simulink model "Appl_HeatFault_CtrlModel"  (R2018b)
settings: configuration reference "CodeConfig_10_ms" (kept outside this file)
undefined symbols (not defined in the file): CAL_CmdOpenTime, CAL_CmdShortTime, CAL_NTCOpenTime, CAL_NTCOverTime, CAL_NTCShortTime, CAL_NTCWaitTime, D_HEATFALUT_CmdOpenLoad, D_HEATFALUT_CmdOpenLoad_W, D_HEATFALUT_CmdShortToGnd, D_HEATFALUT_NtcMax, D_HEATFALUT_NtcMin, D_HEATFALUT_NtcOpenLoad, D_HEATFALUT_NtcShortToGnd, FALSE, TRUE
libraries: DareLib x32, simulink x1
(part 1 of 2)
settings Model: Creator=Administrator  LastModifiedBy=Administrator
settings ConfigSetRef: SourceLocation=Base Workspace

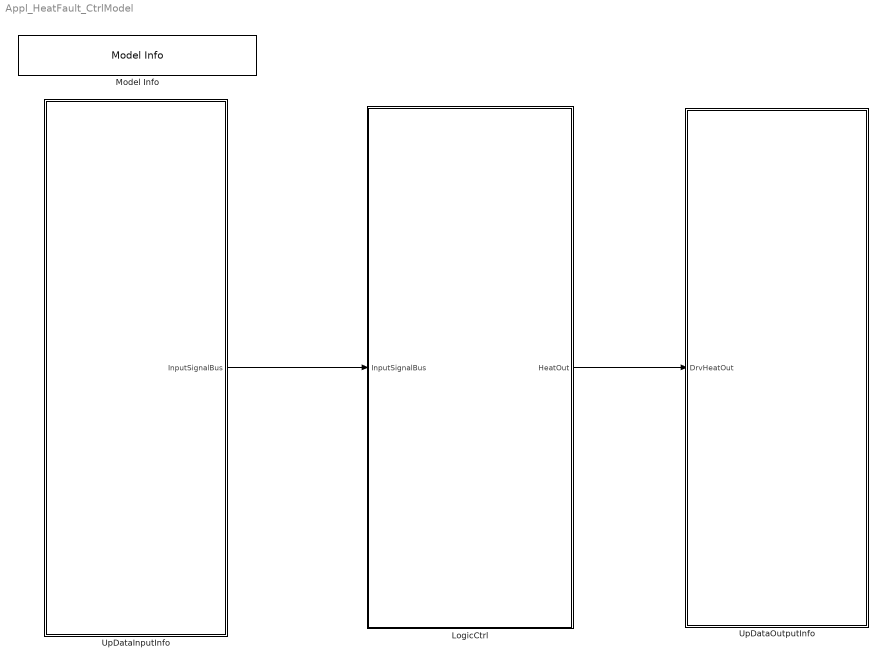
== system Appl_HeatFault_CtrlModel ==
  LogicCtrl : Subsystem  Priority=2  TreatAsAtomicUnit=on
      settings: RTWSystemCode=Nonreusable function  RTWFcnNameOpts=Use subsystem name
  Model Info : simulink/Model-Wide Utilities/Model Info  Frame=on  DisplayStringWithTags=Version：%<ModelVersion>  HorizontalTextAlignment=Center  LeftAlignmentValue=0.5
  UpDataInputInfo : Subsystem  Priority=1  TreatAsAtomicUnit=on
      settings: RTWSystemCode=Nonreusable function  RTWFcnNameOpts=Use subsystem name
  UpDataOutputInfo : Subsystem  Priority=3  TreatAsAtomicUnit=on
      settings: RTWSystemCode=Nonreusable function  RTWFcnNameOpts=Use subsystem name
  wires:
  LogicCtrl/1(HeatOut) -> UpDataOutputInfo/1(DrvHeatOut)
  UpDataInputInfo/1(InputSignalBus) -> LogicCtrl/1(InputSignalBus)

== system Appl_HeatFault_CtrlModel/LogicCtrl ==
  InputSignalBus : Inport
  Bus Selector : BusSelector  OutputSignals=Rte_SignalBus.HeatFalut_D_SimuIndex_DRHeat,Rte_SignalBus.HeatFalut_D_SimuIndex_PAHeat,Rte_SignalBus.HeatFalut_D_SimuIndex_ThirdHeat,Rte_SignalBus.HeatFalut_D_SimuIndex_DRHeatIo,Rte_SignalBus.HeatFalut_D_SimuIndex_PAHeatIo,Rte_SignalBus.HeatFalut_D_SimuIndex_ThirdHeatIo,Rte_SignalBus.HeatFalut_MemIndexDrHeatConfig,Rte_SignalBus.HeatFalut_MemIndexPaHeatConfig,Rte_SignalBus.HeatFalut_MemIndexThirdHeatConfig,Rte_SignalBus.HeatFalut_DrHeatNtcAdc,Rte_SignalBus.HeatFalut_PaHeatNtcAdc,Rte_SignalBus.HeatFalut_ThirdHeatNtcAdc,Rte_SignalBus.HeatFalut_DrHeatIsAdc,Rte_SignalBus.HeatFalut_PaHeatIsAdc,Rte_SignalBus.HeatFalut_ThirdHeatIsAdc,DrFaultType,PaFaultType,ThirdFaultType,Rte_SignalBus.HeatFalut_MemDiagDrHeatFlg,Rte_SignalBus.HeatFalut_MemDiagPaHeatFlg
  HeatDiagnoseCtrl : Subsystem  Description=加热诊断处理
      settings: AttributesFormatString=%<Description>
  MainVent_OutputLvlSts : BusCreator  Inputs=9
  HeatOut : Outport
  wires:
  InputSignalBus/1 -> Bus Selector/1  "InputSignalBus"
  MainVent_OutputLvlSts/1 -> HeatOut/1
  Bus Selector/15 -> HeatDiagnoseCtrl/15(HeatFalut_ThirdHeatIsAdc)  "<HeatFalut_ThirdHeatIsAdc>"
  Bus Selector/14 -> HeatDiagnoseCtrl/14(HeatFalut_PaHeatIsAdc)  "<HeatFalut_PaHeatIsAdc>"
  Bus Selector/13 -> HeatDiagnoseCtrl/13(HeatFalut_DrHeatIsAdc)  "<HeatFalut_DrHeatIsAdc>"
  Bus Selector/12 -> HeatDiagnoseCtrl/12(HeatFalut_ThirdHeatNtcAdc)  "<HeatFalut_ThirdHeatNtcAdc>"
  Bus Selector/11 -> HeatDiagnoseCtrl/11(HeatFalut_PaHeatNtcAdc)  "<HeatFalut_PaHeatNtcAdc>"
  Bus Selector/10 -> HeatDiagnoseCtrl/10(HeatFalut_DrHeatNtcAdc)  "<HeatFalut_DrHeatNtcAdc>"
  Bus Selector/9 -> HeatDiagnoseCtrl/9(HeatFalut_MemIndexThirdHeatConfig)  "<HeatFalut_MemIndexThirdHeatConfig>"
  Bus Selector/8 -> HeatDiagnoseCtrl/8(HeatFalut_MemIndexPaHeatConfig)  "<HeatFalut_MemIndexPaHeatConfig>"
  Bus Selector/7 -> HeatDiagnoseCtrl/7(HeatFalut_MemIndexDrHeatConfig)  "<HeatFalut_MemIndexDrHeatConfig>"
  Bus Selector/6 -> HeatDiagnoseCtrl/6(HeatFalut_D_SimuIndex_ThirdHeatIo)  "<HeatFalut_D_SimuIndex_ThirdHeatIo>"
  Bus Selector/5 -> HeatDiagnoseCtrl/5(HeatFalut_D_SimuIndex_PAHeatIo)  "<HeatFalut_D_SimuIndex_PAHeatIo>"
  Bus Selector/4 -> HeatDiagnoseCtrl/4(HeatFalut_D_SimuIndex_DRHeatIo)  "<HeatFalut_D_SimuIndex_DRHeatIo>"
  Bus Selector/3 -> HeatDiagnoseCtrl/3(HeatFalut_D_SimuIndex_ThirdHeat)  "<HeatFalut_D_SimuIndex_ThirdHeat>"
  Bus Selector/2 -> HeatDiagnoseCtrl/2(HeatFalut_D_SimuIndex_PAHeat)  "<HeatFalut_D_SimuIndex_PAHeat>"
  Bus Selector/1 -> HeatDiagnoseCtrl/1(HeatFalut_D_SimuIndex_DRHeat)  "<HeatFalut_D_SimuIndex_DRHeat>"
  HeatDiagnoseCtrl/1(HeatFault_DRHeatCmdFaultSts) -> MainVent_OutputLvlSts/1
  HeatDiagnoseCtrl/2(HeatFault_PAHeatCmdFaultSts) -> MainVent_OutputLvlSts/2
  HeatDiagnoseCtrl/3(HeatFault_ThirdHeatCmdFaultSts) -> MainVent_OutputLvlSts/3
  HeatDiagnoseCtrl/4(HeatFault_DRHeatNTCFaultSts) -> MainVent_OutputLvlSts/4
  HeatDiagnoseCtrl/5(HeatFault_PAHeatNTCFaultSts) -> MainVent_OutputLvlSts/5
  HeatDiagnoseCtrl/6(HeatFault_ThirdHeatNTCFaultSts) -> MainVent_OutputLvlSts/6
  HeatDiagnoseCtrl/7(HeatFault_DRHeatCmdFaultSts4DTC) -> MainVent_OutputLvlSts/7
  HeatDiagnoseCtrl/8(HeatFault_PAHeatCmdFaultSts4DTC) -> MainVent_OutputLvlSts/8
  HeatDiagnoseCtrl/9(HeatFault_ThirdHeatCmdFaultSts4DTC) -> MainVent_OutputLvlSts/9
  Bus Selector/16 -> HeatDiagnoseCtrl/16(DrFaultType)  "<DrFaultType>"
  Bus Selector/17 -> HeatDiagnoseCtrl/17(PaFaultType)  "<PaFaultType>"
  Bus Selector/18 -> HeatDiagnoseCtrl/18(ThirdFaultType)  "<ThirdFaultType>"
  Bus Selector/19 -> HeatDiagnoseCtrl/19(HeatFalut_MemDiagDrHeatFlg)  "<HeatFalut_MemDiagDrHeatFlg>"
  Bus Selector/20 -> HeatDiagnoseCtrl/20(HeatFalut_MemDiagPaHeatFlg)  "<HeatFalut_MemDiagPaHeatFlg>"

== system Appl_HeatFault_CtrlModel/UpDataInputInfo ==
  InputSignalProcess : Subsystem  Description=数据处理
      settings: AttributesFormatString=%<Description>  RTWSystemCode=Nonreusable function  RTWFcnNameOpts=Use subsystem name
  RTE : Subsystem  Description=接口自动生成  TreatAsAtomicUnit=on
      settings: AttributesFormatString=%<Description>  RTWSystemCode=Nonreusable function  RTWFcnNameOpts=Use subsystem name
  InputSignalBus : Outport
  wires:
  RTE/1(RTE_Signal) -> InputSignalProcess/1(Rte_SignalBus)
  InputSignalProcess/1(InputSignalBus) -> InputSignalBus/1

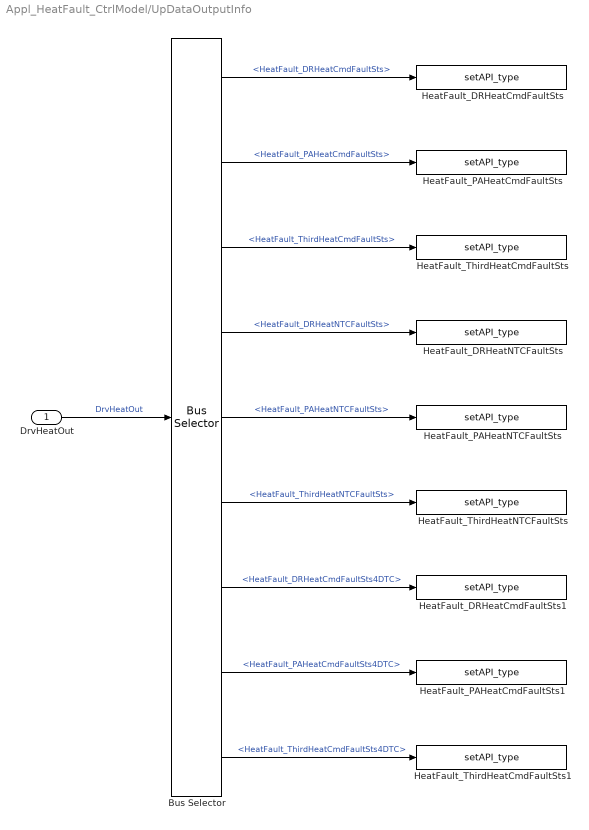
== system Appl_HeatFault_CtrlModel/UpDataOutputInfo ==
  DrvHeatOut : Inport
  Bus Selector : BusSelector  OutputSignals=HeatFault_DRHeatCmdFaultSts,HeatFault_PAHeatCmdFaultSts,HeatFault_ThirdHeatCmdFaultSts,HeatFault_DRHeatNTCFaultSts,HeatFault_PAHeatNTCFaultSts,HeatFault_ThirdHeatNTCFaultSts,HeatFault_DRHeatCmdFaultSts4DTC,HeatFault_PAHeatCmdFaultSts4DTC,HeatFault_ThirdHeatCmdFaultSts4DTC
  HeatFault_DRHeatCmdFaultSts : DareLib/Dare/setAPI_type  g_funcname=Rte_SetVfb_DrHeatCmdFaultSts  g_param=""  g_type=uint8  g_enum=enHeatCmdFault  g_size=-1
      settings: AttributesFormatString=%<g_funcname>  SourceProductName=Dare Library
  HeatFault_DRHeatCmdFaultSts1 : DareLib/Dare/setAPI_type  g_funcname=Rte_SetVfb_DrHeatCmdFaultSts4DTC  g_param=""  g_type=uint8  g_enum=enHeatCmdFault  g_size=-1
      settings: AttributesFormatString=%<g_funcname>  SourceProductName=Dare Library
  HeatFault_DRHeatNTCFaultSts : DareLib/Dare/setAPI_type  g_funcname=Rte_SetVfb_DrHeatNTCFaultSts  g_param=""  g_type=uint8  g_enum=enHeatNtcFault  g_size=-1
      settings: AttributesFormatString=%<g_funcname>  SourceProductName=Dare Library
  HeatFault_PAHeatCmdFaultSts : DareLib/Dare/setAPI_type  g_funcname=Rte_SetVfb_PaHeatCmdFaultSts  g_param=""  g_type=uint8  g_enum=enHeatCmdFault  g_size=-1
      settings: AttributesFormatString=%<g_funcname>  SourceProductName=Dare Library
  HeatFault_PAHeatCmdFaultSts1 : DareLib/Dare/setAPI_type  g_funcname=Rte_SetVfb_PaHeatCmdFaultSts4DTC  g_param=""  g_type=uint8  g_enum=enHeatCmdFault  g_size=-1
      settings: AttributesFormatString=%<g_funcname>  SourceProductName=Dare Library
  HeatFault_PAHeatNTCFaultSts : DareLib/Dare/setAPI_type  g_funcname=Rte_SetVfb_PaHeatNTCFaultSts  g_param=""  g_type=uint8  g_enum=enHeatNtcFault  g_size=-1
      settings: AttributesFormatString=%<g_funcname>  SourceProductName=Dare Library
  HeatFault_ThirdHeatCmdFaultSts : DareLib/Dare/setAPI_type  g_funcname=Rte_SetVfb_ThirdHeatCmdFaultSts  g_param=""  g_type=uint8  g_enum=enHeatCmdFault  g_size=-1
      settings: AttributesFormatString=%<g_funcname>  SourceProductName=Dare Library
  HeatFault_ThirdHeatCmdFaultSts1 : DareLib/Dare/setAPI_type  g_funcname=Rte_SetVfb_ThirdHeatCmdFaultSts4DTC  g_param=""  g_type=uint8  g_enum=enHeatCmdFault  g_size=-1
      settings: AttributesFormatString=%<g_funcname>  SourceProductName=Dare Library
  HeatFault_ThirdHeatNTCFaultSts : DareLib/Dare/setAPI_type  g_funcname=Rte_SetVfb_ThirdHeatNTCFaultSts  g_param=""  g_type=uint8  g_enum=enHeatNtcFault  g_size=-1
      settings: AttributesFormatString=%<g_funcname>  SourceProductName=Dare Library
  wires:
  DrvHeatOut/1 -> Bus Selector/1  "DrvHeatOut"
  Bus Selector/1 -> HeatFault_DRHeatCmdFaultSts/1  "<HeatFault_DRHeatCmdFaultSts>"
  Bus Selector/2 -> HeatFault_PAHeatCmdFaultSts/1  "<HeatFault_PAHeatCmdFaultSts>"
  Bus Selector/3 -> HeatFault_ThirdHeatCmdFaultSts/1  "<HeatFault_ThirdHeatCmdFaultSts>"
  Bus Selector/4 -> HeatFault_DRHeatNTCFaultSts/1  "<HeatFault_DRHeatNTCFaultSts>"
  Bus Selector/5 -> HeatFault_PAHeatNTCFaultSts/1  "<HeatFault_PAHeatNTCFaultSts>"
  Bus Selector/6 -> HeatFault_ThirdHeatNTCFaultSts/1  "<HeatFault_ThirdHeatNTCFaultSts>"
  Bus Selector/7 -> HeatFault_DRHeatCmdFaultSts1/1  "<HeatFault_DRHeatCmdFaultSts4DTC>"
  Bus Selector/8 -> HeatFault_PAHeatCmdFaultSts1/1  "<HeatFault_PAHeatCmdFaultSts4DTC>"
  Bus Selector/9 -> HeatFault_ThirdHeatCmdFaultSts1/1  "<HeatFault_ThirdHeatCmdFaultSts4DTC>"

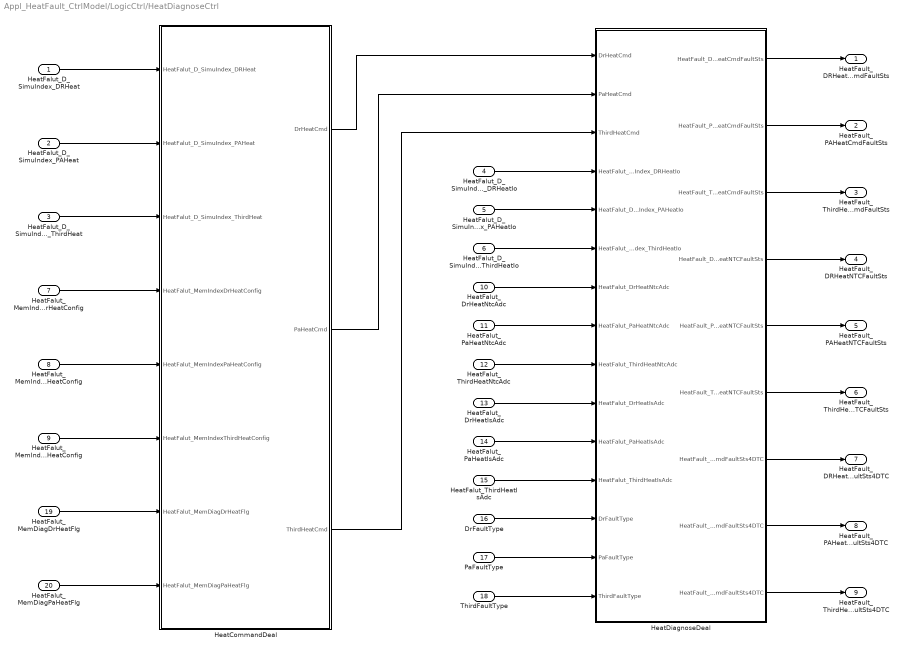
== system Appl_HeatFault_CtrlModel/LogicCtrl/HeatDiagnoseCtrl ==
  HeatFalut_D_SimuIndex_DRHeat : Inport
  HeatFalut_D_SimuIndex_PAHeat : Inport  Port=2
  HeatFalut_D_SimuIndex_ThirdHeat : Inport  Port=3
  HeatFalut_D_SimuIndex_DRHeatIo : Inport  Port=4
  HeatFalut_D_SimuIndex_PAHeatIo : Inport  Port=5
  HeatFalut_D_SimuIndex_ThirdHeatIo : Inport  Port=6
  HeatFalut_MemIndexDrHeatConfig : Inport  Port=7
  HeatFalut_MemIndexPaHeatConfig : Inport  Port=8
  HeatFalut_MemIndexThirdHeatConfig : Inport  Port=9
  HeatFalut_DrHeatNtcAdc : Inport  Port=10
  HeatFalut_PaHeatNtcAdc : Inport  Port=11
  HeatFalut_ThirdHeatNtcAdc : Inport  Port=12
  HeatFalut_DrHeatIsAdc : Inport  Port=13
  HeatFalut_PaHeatIsAdc : Inport  Port=14
  HeatFalut_ThirdHeatIsAdc : Inport  Port=15
  DrFaultType : Inport  Port=16
  PaFaultType : Inport  Port=17
  ThirdFaultType : Inport  Port=18
  HeatFalut_MemDiagDrHeatFlg : Inport  Port=19
  HeatFalut_MemDiagPaHeatFlg : Inport  Port=20
  HeatCommandDeal : Stateflow chart  TreatAsAtomicUnit=on
  HeatDiagnoseDeal : Stateflow chart  TreatAsAtomicUnit=on
  HeatFault_DRHeatCmdFaultSts : Outport
  HeatFault_PAHeatCmdFaultSts : Outport  Port=2
  HeatFault_ThirdHeatCmdFaultSts : Outport  Port=3
  HeatFault_DRHeatNTCFaultSts : Outport  Port=4
  HeatFault_PAHeatNTCFaultSts : Outport  Port=5
  HeatFault_ThirdHeatNTCFaultSts : Outport  Port=6
  HeatFault_DRHeatCmdFaultSts4DTC : Outport  Port=7
  HeatFault_PAHeatCmdFaultSts4DTC : Outport  Port=8
  HeatFault_ThirdHeatCmdFaultSts4DTC : Outport  Port=9
  wires:
  HeatDiagnoseDeal/3(HeatFault_ThirdHeatCmdFaultSts) -> HeatFault_ThirdHeatCmdFaultSts/1
  HeatDiagnoseDeal/2(HeatFault_PAHeatCmdFaultSts) -> HeatFault_PAHeatCmdFaultSts/1
  HeatDiagnoseDeal/4(HeatFault_DRHeatNTCFaultSts) -> HeatFault_DRHeatNTCFaultSts/1
  HeatDiagnoseDeal/1(HeatFault_DRHeatCmdFaultSts) -> HeatFault_DRHeatCmdFaultSts/1
  HeatDiagnoseDeal/5(HeatFault_PAHeatNTCFaultSts) -> HeatFault_PAHeatNTCFaultSts/1
  HeatDiagnoseDeal/6(HeatFault_ThirdHeatNTCFaultSts) -> HeatFault_ThirdHeatNTCFaultSts/1
  HeatFalut_D_SimuIndex_DRHeat/1 -> HeatCommandDeal/1(HeatFalut_D_SimuIndex_DRHeat)
  HeatFalut_D_SimuIndex_PAHeat/1 -> HeatCommandDeal/2(HeatFalut_D_SimuIndex_PAHeat)
  HeatFalut_MemIndexDrHeatConfig/1 -> HeatCommandDeal/4(HeatFalut_MemIndexDrHeatConfig)
  HeatFalut_D_SimuIndex_ThirdHeat/1 -> HeatCommandDeal/3(HeatFalut_D_SimuIndex_ThirdHeat)
  HeatFalut_MemIndexPaHeatConfig/1 -> HeatCommandDeal/5(HeatFalut_MemIndexPaHeatConfig)
  HeatFalut_MemIndexThirdHeatConfig/1 -> HeatCommandDeal/6(HeatFalut_MemIndexThirdHeatConfig)
  HeatCommandDeal/1(DrHeatCmd) -> HeatDiagnoseDeal/1(DrHeatCmd)
  HeatCommandDeal/2(PaHeatCmd) -> HeatDiagnoseDeal/2(PaHeatCmd)
  HeatCommandDeal/3(ThirdHeatCmd) -> HeatDiagnoseDeal/3(ThirdHeatCmd)
  HeatFalut_D_SimuIndex_DRHeatIo/1 -> HeatDiagnoseDeal/4(HeatFalut_D_SimuIndex_DRHeatIo)
  HeatFalut_D_SimuIndex_PAHeatIo/1 -> HeatDiagnoseDeal/5(HeatFalut_D_SimuIndex_PAHeatIo)
  HeatFalut_D_SimuIndex_ThirdHeatIo/1 -> HeatDiagnoseDeal/6(HeatFalut_D_SimuIndex_ThirdHeatIo)
  HeatFalut_ThirdHeatIsAdc/1 -> HeatDiagnoseDeal/12(HeatFalut_ThirdHeatIsAdc)
  HeatFalut_PaHeatIsAdc/1 -> HeatDiagnoseDeal/11(HeatFalut_PaHeatIsAdc)
  HeatFalut_DrHeatIsAdc/1 -> HeatDiagnoseDeal/10(HeatFalut_DrHeatIsAdc)
  HeatFalut_ThirdHeatNtcAdc/1 -> HeatDiagnoseDeal/9(HeatFalut_ThirdHeatNtcAdc)
  HeatFalut_PaHeatNtcAdc/1 -> HeatDiagnoseDeal/8(HeatFalut_PaHeatNtcAdc)
  HeatFalut_DrHeatNtcAdc/1 -> HeatDiagnoseDeal/7(HeatFalut_DrHeatNtcAdc)
  HeatDiagnoseDeal/7(HeatFault_DRHeatCmdFaultSts4DTC) -> HeatFault_DRHeatCmdFaultSts4DTC/1
  HeatDiagnoseDeal/8(HeatFault_PAHeatCmdFaultSts4DTC) -> HeatFault_PAHeatCmdFaultSts4DTC/1
  HeatDiagnoseDeal/9(HeatFault_ThirdHeatCmdFaultSts4DTC) -> HeatFault_ThirdHeatCmdFaultSts4DTC/1
  DrFaultType/1 -> HeatDiagnoseDeal/13(DrFaultType)
  PaFaultType/1 -> HeatDiagnoseDeal/14(PaFaultType)
  ThirdFaultType/1 -> HeatDiagnoseDeal/15(ThirdFaultType)
  HeatFalut_MemDiagPaHeatFlg/1 -> HeatCommandDeal/8(HeatFalut_MemDiagPaHeatFlg)
  HeatFalut_MemDiagDrHeatFlg/1 -> HeatCommandDeal/7(HeatFalut_MemDiagDrHeatFlg)

== system Appl_HeatFault_CtrlModel/UpDataInputInfo/InputSignalProcess ==
  Rte_SignalBus : Inport
  Bus Creator : BusCreator  Inputs=4
  Bus Selector : BusSelector  OutputSignals=HeatFalut_DrCmdShortGND,HeatFalut_PaCmdShortGND,HeatFalut_3rdCmdShortGND,HeatFalut_DrCmdOpenload,HeatFalut_PaCmdOpenload,HeatFalut_3rdCmdOpenload
  CMD_Process : Subsystem  Description=CMD诊断DTC处理（确认当前CMD有哪个DTC）
      settings: AttributesFormatString=%<Description>
  InputSignalBus : Outport
  wires:
  Bus Creator/1 -> InputSignalBus/1
  Rte_SignalBus/1 -> Bus Selector/1, Bus Creator/1  "Rte_SignalBus"
  Bus Selector/1 -> CMD_Process/1(HeatFalut_DrCmdShortGND)  "<HeatFalut_DrCmdShortGND>"
  Bus Selector/2 -> CMD_Process/2(HeatFalut_PaCmdShortGND)  "<HeatFalut_PaCmdShortGND>"
  Bus Selector/3 -> CMD_Process/3(HeatFalut_3rdCmdShortGND)  "<HeatFalut_3rdCmdShortGND>"
  Bus Selector/4 -> CMD_Process/4(HeatFalut_DrCmdOpenload)  "<HeatFalut_DrCmdOpenload>"
  Bus Selector/5 -> CMD_Process/5(HeatFalut_PaCmdOpenload)  "<HeatFalut_PaCmdOpenload>"
  Bus Selector/6 -> CMD_Process/6(HeatFalut_3rdCmdOpenload)  "<HeatFalut_3rdCmdOpenload>"
  CMD_Process/1(DrFaultType) -> Bus Creator/2
  CMD_Process/2(PaFaultType) -> Bus Creator/3
  CMD_Process/3(ThirdFaultType) -> Bus Creator/4

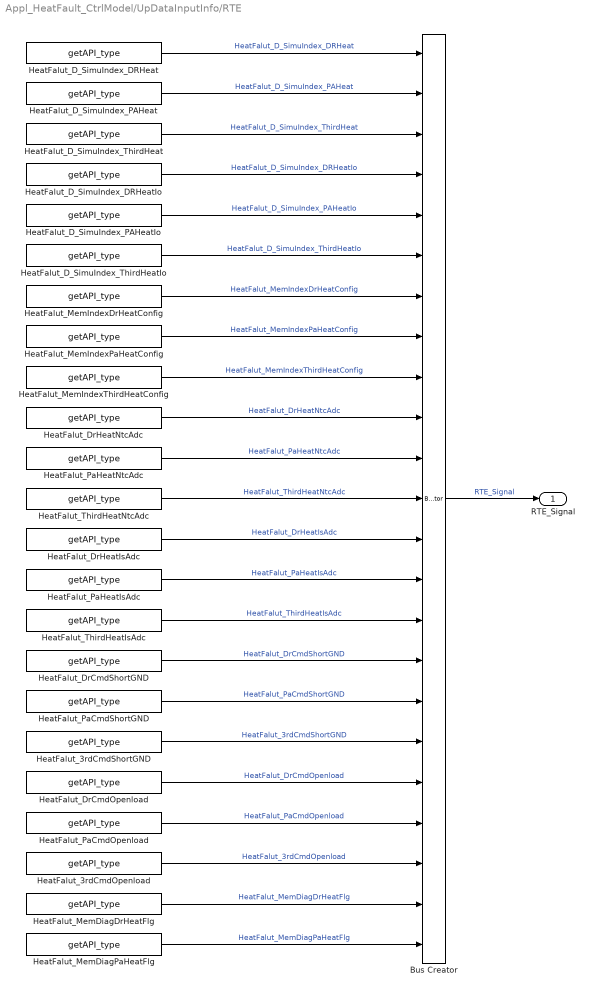
== system Appl_HeatFault_CtrlModel/UpDataInputInfo/RTE ==
  Bus Creator : BusCreator  Inputs=23
  HeatFalut_3rdCmdOpenload : DareLib/Dare/getAPI_type  g_funcname=Diag_ReadDtcTestFailFlag  g_param=D_DTC_3rdHeatOutputOp  g_type=uint8  g_size=-1
      settings: AttributesFormatString=%<g_funcname>  SourceProductName=Dare Library
  HeatFalut_3rdCmdShortGND : DareLib/Dare/getAPI_type  g_funcname=Diag_ReadDtcTestFailFlag  g_param=D_DTC_3rdHeatOutputGS  g_type=uint8  g_size=-1
      settings: AttributesFormatString=%<g_funcname>  SourceProductName=Dare Library
  HeatFalut_D_SimuIndex_DRHeat : DareLib/Dare/getAPI_type  g_funcname=Rte_GetVfb_DrHeat  g_param=""  g_type=uint8  g_enum=enHeatLvlSts  g_size=-1
      settings: AttributesFormatString=%<g_funcname>  SourceProductName=Dare Library
  HeatFalut_D_SimuIndex_DRHeatIo : DareLib/Dare/getAPI_type  g_funcname=Rte_GetVfb_DrHeatIo  g_param=""  g_type=uint8  g_enum=enHeatIoSts  g_size=-1
      settings: AttributesFormatString=%<g_funcname>  SourceProductName=Dare Library
  HeatFalut_D_SimuIndex_PAHeat : DareLib/Dare/getAPI_type  g_funcname=Rte_GetVfb_PaHeat  g_param=""  g_type=uint8  g_enum=enHeatLvlSts  g_size=-1
      settings: AttributesFormatString=%<g_funcname>  SourceProductName=Dare Library
  HeatFalut_D_SimuIndex_PAHeatIo : DareLib/Dare/getAPI_type  g_funcname=Rte_GetVfb_PaHeatIo  g_param=""  g_type=uint8  g_enum=enHeatIoSts  g_size=-1
      settings: AttributesFormatString=%<g_funcname>  SourceProductName=Dare Library
  HeatFalut_D_SimuIndex_ThirdHeat : DareLib/Dare/getAPI_type  g_funcname=Rte_GetVfb_ThirdHeat  g_param=""  g_type=uint8  g_enum=enHeatLvlSts  g_size=-1
      settings: AttributesFormatString=%<g_funcname>  SourceProductName=Dare Library
  HeatFalut_D_SimuIndex_ThirdHeatIo : DareLib/Dare/getAPI_type  g_funcname=Rte_GetVfb_ThirdHeatIo  g_param=""  g_type=uint8  g_enum=enHeatIoSts  g_size=-1
      settings: AttributesFormatString=%<g_funcname>  SourceProductName=Dare Library
  HeatFalut_DrCmdOpenload : DareLib/Dare/getAPI_type  g_funcname=Diag_ReadDtcTestFailFlag  g_param=D_DTC_DrHeatOutputOp  g_type=uint8  g_size=-1
      settings: AttributesFormatString=%<g_funcname>  SourceProductName=Dare Library
  HeatFalut_DrCmdShortGND : DareLib/Dare/getAPI_type  g_funcname=Diag_ReadDtcTestFailFlag  g_param=D_DTC_DrHeatOutputGS  g_type=uint8  g_size=-1
      settings: AttributesFormatString=%<g_funcname>  SourceProductName=Dare Library
  HeatFalut_DrHeatIsAdc : DareLib/Dare/getAPI_type  g_funcname=Ecual_AdcGetChlStatus  g_param=enADC_DrHeaterIS  g_type=uint16  g_size=-1
      settings: AttributesFormatString=%<g_funcname>  SourceProductName=Dare Library
  HeatFalut_DrHeatNtcAdc : DareLib/Dare/getAPI_type  g_funcname=Ecual_AdcGetChlStatus  g_param=enADC_DrHeaterNTC  g_type=uint16  g_size=-1
      settings: AttributesFormatString=%<g_funcname>  SourceProductName=Dare Library
  HeatFalut_MemDiagDrHeatFlg : DareLib/Dare/getAPI_type  g_funcname=Srvl_GetMemIndexDataU8  g_param=EN_MemIndex_DrHeatFlg  g_type=uint8  g_size=-1
      settings: AttributesFormatString=%<g_funcname>  SourceProductName=Dare Library
  HeatFalut_MemDiagPaHeatFlg : DareLib/Dare/getAPI_type  g_funcname=Srvl_GetMemIndexDataU8  g_param=EN_MemIndex_PaHeatFlg  g_type=uint8  g_size=-1
      settings: AttributesFormatString=%<g_funcname>  SourceProductName=Dare Library
  HeatFalut_MemIndexDrHeatConfig : DareLib/Dare/getAPI_type  g_funcname=Rte_GetVfb_DrHeatEnable  g_param=""  g_type=uint8  g_enum=enHeatIoSts  g_size=-1
      settings: AttributesFormatString=%<g_funcname>  SourceProductName=Dare Library
  HeatFalut_MemIndexPaHeatConfig : DareLib/Dare/getAPI_type  g_funcname=Rte_GetVfb_SecondHeatEnable  g_param=""  g_type=uint8  g_size=-1
      settings: AttributesFormatString=%<g_funcname>  SourceProductName=Dare Library
  HeatFalut_MemIndexThirdHeatConfig : DareLib/Dare/getAPI_type  g_funcname=Rte_GetVfb_ThirdHeatEnable  g_param=""  g_type=uint8  g_size=-1
      settings: AttributesFormatString=%<g_funcname>  SourceProductName=Dare Library
  HeatFalut_PaCmdOpenload : DareLib/Dare/getAPI_type  g_funcname=Diag_ReadDtcTestFailFlag  g_param=D_DTC_PaHeatOutputOp  g_type=uint8  g_size=-1
      settings: AttributesFormatString=%<g_funcname>  SourceProductName=Dare Library
  HeatFalut_PaCmdShortGND : DareLib/Dare/getAPI_type  g_funcname=Diag_ReadDtcTestFailFlag  g_param=D_DTC_PaHeatOutputGS  g_type=uint8  g_size=-1
      settings: AttributesFormatString=%<g_funcname>  SourceProductName=Dare Library
  HeatFalut_PaHeatIsAdc : DareLib/Dare/getAPI_type  g_funcname=Ecual_AdcGetChlStatus  g_param=enADC_PaHeaterIS  g_type=uint16  g_size=-1
      settings: AttributesFormatString=%<g_funcname>  SourceProductName=Dare Library
  HeatFalut_PaHeatNtcAdc : DareLib/Dare/getAPI_type  g_funcname=Ecual_AdcGetChlStatus  g_param=enADC_PaHeaterNTC  g_type=uint16  g_size=-1
      settings: AttributesFormatString=%<g_funcname>  SourceProductName=Dare Library
  HeatFalut_ThirdHeatIsAdc : DareLib/Dare/getAPI_type  g_funcname=Ecual_AdcGetChlStatus  g_param=enADC_SteerHeaterIS  g_type=uint16  g_size=-1
      settings: AttributesFormatString=%<g_funcname>  SourceProductName=Dare Library
  HeatFalut_ThirdHeatNtcAdc : DareLib/Dare/getAPI_type  g_funcname=Ecual_AdcGetChlStatus  g_param=enADC_SteerHeaterNTC  g_type=uint16  g_size=-1
      settings: AttributesFormatString=%<g_funcname>  SourceProductName=Dare Library
  RTE_Signal : Outport
  wires:
  Bus Creator/1 -> RTE_Signal/1  "RTE_Signal"
  HeatFalut_D_SimuIndex_DRHeat/1 -> Bus Creator/1  "HeatFalut_D_SimuIndex_DRHeat"
  HeatFalut_D_SimuIndex_PAHeat/1 -> Bus Creator/2  "HeatFalut_D_SimuIndex_PAHeat"
  HeatFalut_D_SimuIndex_ThirdHeat/1 -> Bus Creator/3  "HeatFalut_D_SimuIndex_ThirdHeat"
  HeatFalut_D_SimuIndex_DRHeatIo/1 -> Bus Creator/4  "HeatFalut_D_SimuIndex_DRHeatIo"
  HeatFalut_D_SimuIndex_PAHeatIo/1 -> Bus Creator/5  "HeatFalut_D_SimuIndex_PAHeatIo"
  HeatFalut_D_SimuIndex_ThirdHeatIo/1 -> Bus Creator/6  "HeatFalut_D_SimuIndex_ThirdHeatIo"
  HeatFalut_MemIndexDrHeatConfig/1 -> Bus Creator/7  "HeatFalut_MemIndexDrHeatConfig"
  HeatFalut_MemIndexPaHeatConfig/1 -> Bus Creator/8  "HeatFalut_MemIndexPaHeatConfig"
  HeatFalut_MemIndexThirdHeatConfig/1 -> Bus Creator/9  "HeatFalut_MemIndexThirdHeatConfig"
  HeatFalut_DrHeatNtcAdc/1 -> Bus Creator/10  "HeatFalut_DrHeatNtcAdc"
  HeatFalut_PaHeatNtcAdc/1 -> Bus Creator/11  "HeatFalut_PaHeatNtcAdc"
  HeatFalut_ThirdHeatNtcAdc/1 -> Bus Creator/12  "HeatFalut_ThirdHeatNtcAdc"
  HeatFalut_DrHeatIsAdc/1 -> Bus Creator/13  "HeatFalut_DrHeatIsAdc"
  HeatFalut_PaHeatIsAdc/1 -> Bus Creator/14  "HeatFalut_PaHeatIsAdc"
  HeatFalut_ThirdHeatIsAdc/1 -> Bus Creator/15  "HeatFalut_ThirdHeatIsAdc"
  HeatFalut_DrCmdShortGND/1 -> Bus Creator/16  "HeatFalut_DrCmdShortGND"
  HeatFalut_PaCmdShortGND/1 -> Bus Creator/17  "HeatFalut_PaCmdShortGND"
  HeatFalut_3rdCmdShortGND/1 -> Bus Creator/18  "HeatFalut_3rdCmdShortGND"
  HeatFalut_DrCmdOpenload/1 -> Bus Creator/19  "HeatFalut_DrCmdOpenload"
  HeatFalut_PaCmdOpenload/1 -> Bus Creator/20  "HeatFalut_PaCmdOpenload"
  HeatFalut_3rdCmdOpenload/1 -> Bus Creator/21  "HeatFalut_3rdCmdOpenload"
  HeatFalut_MemDiagDrHeatFlg/1 -> Bus Creator/22  "HeatFalut_MemDiagDrHeatFlg"
  HeatFalut_MemDiagPaHeatFlg/1 -> Bus Creator/23  "HeatFalut_MemDiagPaHeatFlg"

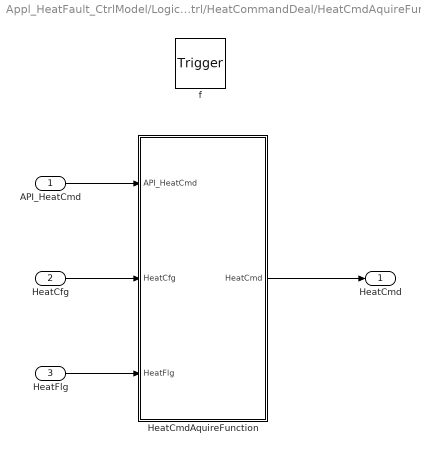
== system Appl_HeatFault_CtrlModel/LogicCtrl/HeatDiagnoseCtrl/HeatCommandDeal/HeatCmdAquireFunction ==
  API_HeatCmd : Inport
  HeatCfg : Inport  Port=2
  HeatFlg : Inport  Port=3
  f : TriggerPort  TriggerType=function-call  VariantControl=(inherit)
      settings: CopyFcn=Stateflow.SLINSF.SimulinkMan.removeBlockPreDeleteFcn  PreDeleteFcn=Stateflow.SLINSF.SimulinkMan.unsafePredeleteFcn
  HeatCmdAquireFunction : Stateflow chart  TreatAsAtomicUnit=on
  HeatCmd : Outport
  wires:
  HeatCfg/1 -> HeatCmdAquireFunction/2(HeatCfg)
  API_HeatCmd/1 -> HeatCmdAquireFunction/1(API_HeatCmd)
  HeatCmdAquireFunction/1(HeatCmd) -> HeatCmd/1
  HeatFlg/1 -> HeatCmdAquireFunction/3(HeatFlg)

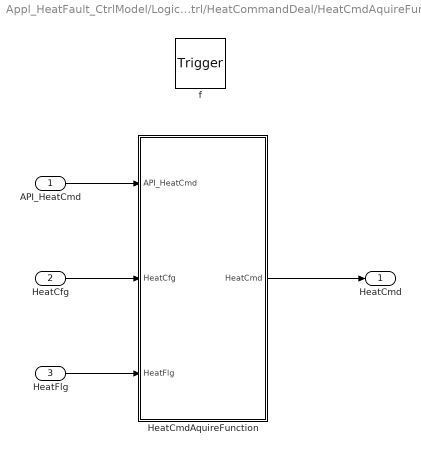
== system Appl_HeatFault_CtrlModel/LogicCtrl/HeatDiagnoseCtrl/HeatCommandDeal/HeatCmdAquireFunction1 ==
  API_HeatCmd : Inport
  HeatCfg : Inport  Port=2
  HeatFlg : Inport  Port=3
  f : TriggerPort  TriggerType=function-call  VariantControl=(inherit)
      settings: CopyFcn=Stateflow.SLINSF.SimulinkMan.removeBlockPreDeleteFcn  PreDeleteFcn=Stateflow.SLINSF.SimulinkMan.unsafePredeleteFcn
  HeatCmdAquireFunction : Stateflow chart  TreatAsAtomicUnit=on
  HeatCmd : Outport
  wires:
  HeatCfg/1 -> HeatCmdAquireFunction/2(HeatCfg)
  API_HeatCmd/1 -> HeatCmdAquireFunction/1(API_HeatCmd)
  HeatCmdAquireFunction/1(HeatCmd) -> HeatCmd/1
  HeatFlg/1 -> HeatCmdAquireFunction/3(HeatFlg)

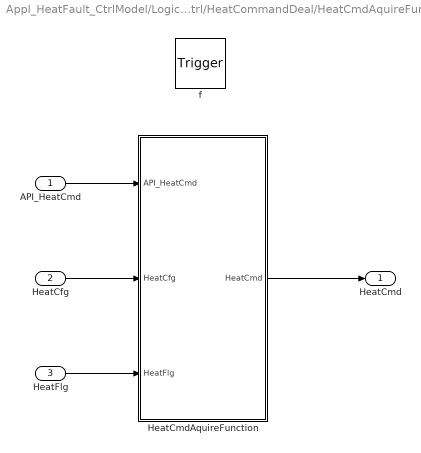
== system Appl_HeatFault_CtrlModel/LogicCtrl/HeatDiagnoseCtrl/HeatCommandDeal/HeatCmdAquireFunction2 ==
  API_HeatCmd : Inport
  HeatCfg : Inport  Port=2
  HeatFlg : Inport  Port=3
  f : TriggerPort  TriggerType=function-call  VariantControl=(inherit)
      settings: CopyFcn=Stateflow.SLINSF.SimulinkMan.removeBlockPreDeleteFcn  PreDeleteFcn=Stateflow.SLINSF.SimulinkMan.unsafePredeleteFcn
  HeatCmdAquireFunction : Stateflow chart  TreatAsAtomicUnit=on
  HeatCmd : Outport
  wires:
  HeatCfg/1 -> HeatCmdAquireFunction/2(HeatCfg)
  API_HeatCmd/1 -> HeatCmdAquireFunction/1(API_HeatCmd)
  HeatCmdAquireFunction/1(HeatCmd) -> HeatCmd/1
  HeatFlg/1 -> HeatCmdAquireFunction/3(HeatFlg)

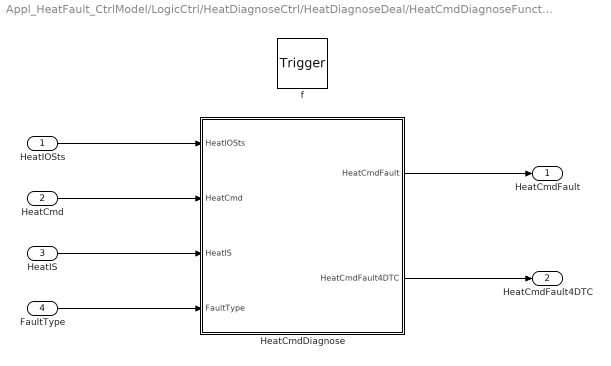
== system Appl_HeatFault_CtrlModel/LogicCtrl/HeatDiagnoseCtrl/HeatDiagnoseDeal/HeatCmdDiagnoseFunction ==
  HeatIOSts : Inport
  HeatCmd : Inport  Port=2
  HeatIS : Inport  Port=3
  FaultType : Inport  Port=4
  f : TriggerPort  TriggerType=function-call  VariantControl=(inherit)
      settings: CopyFcn=Stateflow.SLINSF.SimulinkMan.removeBlockPreDeleteFcn  PreDeleteFcn=Stateflow.SLINSF.SimulinkMan.unsafePredeleteFcn
  HeatCmdDiagnose : Stateflow chart  TreatAsAtomicUnit=on
  HeatCmdFault : Outport
  HeatCmdFault4DTC : Outport  Port=2
  wires:
  FaultType/1 -> HeatCmdDiagnose/4(FaultType)
  HeatIOSts/1 -> HeatCmdDiagnose/1(HeatIOSts)
  HeatCmdDiagnose/2(HeatCmdFault4DTC) -> HeatCmdFault4DTC/1
  HeatCmd/1 -> HeatCmdDiagnose/2(HeatCmd)
  HeatCmdDiagnose/1(HeatCmdFault) -> HeatCmdFault/1
  HeatIS/1 -> HeatCmdDiagnose/3(HeatIS)

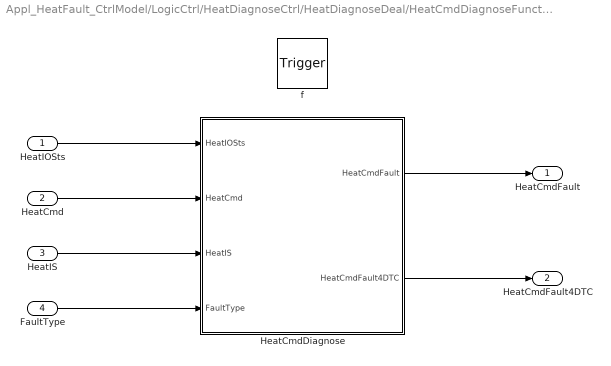
== system Appl_HeatFault_CtrlModel/LogicCtrl/HeatDiagnoseCtrl/HeatDiagnoseDeal/HeatCmdDiagnoseFunction1 ==
  HeatIOSts : Inport
  HeatCmd : Inport  Port=2
  HeatIS : Inport  Port=3
  FaultType : Inport  Port=4
  f : TriggerPort  TriggerType=function-call  VariantControl=(inherit)
      settings: CopyFcn=Stateflow.SLINSF.SimulinkMan.removeBlockPreDeleteFcn  PreDeleteFcn=Stateflow.SLINSF.SimulinkMan.unsafePredeleteFcn
  HeatCmdDiagnose : Stateflow chart  TreatAsAtomicUnit=on
  HeatCmdFault : Outport
  HeatCmdFault4DTC : Outport  Port=2
  wires:
  FaultType/1 -> HeatCmdDiagnose/4(FaultType)
  HeatIOSts/1 -> HeatCmdDiagnose/1(HeatIOSts)
  HeatCmdDiagnose/2(HeatCmdFault4DTC) -> HeatCmdFault4DTC/1
  HeatCmd/1 -> HeatCmdDiagnose/2(HeatCmd)
  HeatCmdDiagnose/1(HeatCmdFault) -> HeatCmdFault/1
  HeatIS/1 -> HeatCmdDiagnose/3(HeatIS)

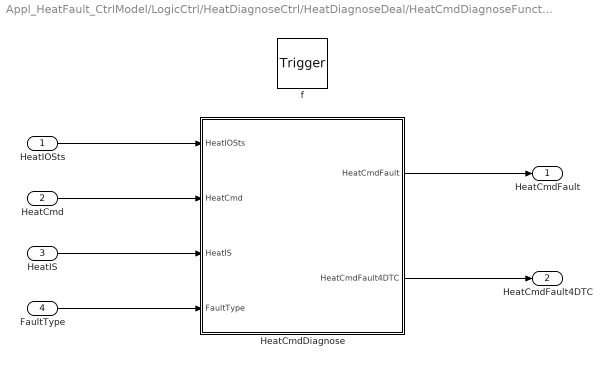
== system Appl_HeatFault_CtrlModel/LogicCtrl/HeatDiagnoseCtrl/HeatDiagnoseDeal/HeatCmdDiagnoseFunction2 ==
  HeatIOSts : Inport
  HeatCmd : Inport  Port=2
  HeatIS : Inport  Port=3
  FaultType : Inport  Port=4
  f : TriggerPort  TriggerType=function-call  VariantControl=(inherit)
      settings: CopyFcn=Stateflow.SLINSF.SimulinkMan.removeBlockPreDeleteFcn  PreDeleteFcn=Stateflow.SLINSF.SimulinkMan.unsafePredeleteFcn
  HeatCmdDiagnose : Stateflow chart  TreatAsAtomicUnit=on
  HeatCmdFault : Outport
  HeatCmdFault4DTC : Outport  Port=2
  wires:
  FaultType/1 -> HeatCmdDiagnose/4(FaultType)
  HeatIOSts/1 -> HeatCmdDiagnose/1(HeatIOSts)
  HeatCmdDiagnose/2(HeatCmdFault4DTC) -> HeatCmdFault4DTC/1
  HeatCmd/1 -> HeatCmdDiagnose/2(HeatCmd)
  HeatCmdDiagnose/1(HeatCmdFault) -> HeatCmdFault/1
  HeatIS/1 -> HeatCmdDiagnose/3(HeatIS)

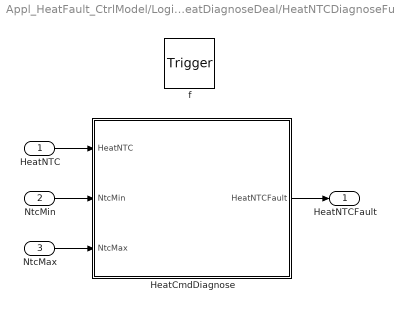
== system Appl_HeatFault_CtrlModel/LogicCtrl/HeatDiagnoseCtrl/HeatDiagnoseDeal/HeatNTCDiagnoseFunction ==
  HeatNTC : Inport
  NtcMin : Inport  Port=2
  NtcMax : Inport  Port=3
  f : TriggerPort  TriggerType=function-call  VariantControl=(inherit)
      settings: CopyFcn=Stateflow.SLINSF.SimulinkMan.removeBlockPreDeleteFcn  PreDeleteFcn=Stateflow.SLINSF.SimulinkMan.unsafePredeleteFcn
  HeatCmdDiagnose : Stateflow chart  TreatAsAtomicUnit=on
  HeatNTCFault : Outport
  wires:
  HeatNTC/1 -> HeatCmdDiagnose/1(HeatNTC)
  HeatCmdDiagnose/1(HeatNTCFault) -> HeatNTCFault/1
  NtcMin/1 -> HeatCmdDiagnose/2(NtcMin)
  NtcMax/1 -> HeatCmdDiagnose/3(NtcMax)

== system Appl_HeatFault_CtrlModel/LogicCtrl/HeatDiagnoseCtrl/HeatDiagnoseDeal/HeatNTCDiagnoseFunction1 ==
  HeatNTC : Inport
  NtcMin : Inport  Port=2
  NtcMax : Inport  Port=3
  f : TriggerPort  TriggerType=function-call  VariantControl=(inherit)
      settings: CopyFcn=Stateflow.SLINSF.SimulinkMan.removeBlockPreDeleteFcn  PreDeleteFcn=Stateflow.SLINSF.SimulinkMan.unsafePredeleteFcn
  HeatCmdDiagnose : Stateflow chart  TreatAsAtomicUnit=on
  HeatNTCFault : Outport
  wires:
  HeatNTC/1 -> HeatCmdDiagnose/1(HeatNTC)
  HeatCmdDiagnose/1(HeatNTCFault) -> HeatNTCFault/1
  NtcMin/1 -> HeatCmdDiagnose/2(NtcMin)
  NtcMax/1 -> HeatCmdDiagnose/3(NtcMax)

== system Appl_HeatFault_CtrlModel/LogicCtrl/HeatDiagnoseCtrl/HeatDiagnoseDeal/HeatNTCDiagnoseFunction2 ==
  HeatNTC : Inport
  NtcMin : Inport  Port=2
  NtcMax : Inport  Port=3
  f : TriggerPort  TriggerType=function-call  VariantControl=(inherit)
      settings: CopyFcn=Stateflow.SLINSF.SimulinkMan.removeBlockPreDeleteFcn  PreDeleteFcn=Stateflow.SLINSF.SimulinkMan.unsafePredeleteFcn
  HeatCmdDiagnose : Stateflow chart  TreatAsAtomicUnit=on
  HeatNTCFault : Outport
  wires:
  HeatNTC/1 -> HeatCmdDiagnose/1(HeatNTC)
  HeatCmdDiagnose/1(HeatNTCFault) -> HeatNTCFault/1
  NtcMin/1 -> HeatCmdDiagnose/2(NtcMin)
  NtcMax/1 -> HeatCmdDiagnose/3(NtcMax)

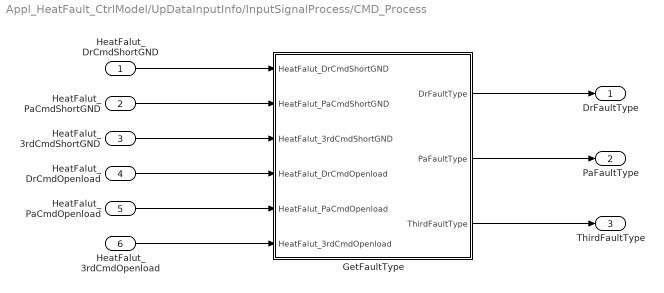
== system Appl_HeatFault_CtrlModel/UpDataInputInfo/InputSignalProcess/CMD_Process ==
  HeatFalut_DrCmdShortGND : Inport
  HeatFalut_PaCmdShortGND : Inport  Port=2
  HeatFalut_3rdCmdShortGND : Inport  Port=3
  HeatFalut_DrCmdOpenload : Inport  Port=4
  HeatFalut_PaCmdOpenload : Inport  Port=5
  HeatFalut_3rdCmdOpenload : Inport  Port=6
  GetFaultType : Stateflow chart  TreatAsAtomicUnit=on
  DrFaultType : Outport
  PaFaultType : Outport  Port=2
  ThirdFaultType : Outport  Port=3
  wires:
  GetFaultType/1(DrFaultType) -> DrFaultType/1
  HeatFalut_DrCmdShortGND/1 -> GetFaultType/1(HeatFalut_DrCmdShortGND)
  HeatFalut_PaCmdShortGND/1 -> GetFaultType/2(HeatFalut_PaCmdShortGND)
  HeatFalut_3rdCmdShortGND/1 -> GetFaultType/3(HeatFalut_3rdCmdShortGND)
  HeatFalut_DrCmdOpenload/1 -> GetFaultType/4(HeatFalut_DrCmdOpenload)
  HeatFalut_PaCmdOpenload/1 -> GetFaultType/5(HeatFalut_PaCmdOpenload)
  HeatFalut_3rdCmdOpenload/1 -> GetFaultType/6(HeatFalut_3rdCmdOpenload)
  GetFaultType/2(PaFaultType) -> PaFaultType/1
  GetFaultType/3(ThirdFaultType) -> ThirdFaultType/1

== system Appl_HeatFault_CtrlModel/UpDataInputInfo/InputSignalProcess/CMD_Process/GetFaultType/getFaultType ==
  ShortGND : Inport
  Openload : Inport  Port=2
  f : TriggerPort  TriggerType=function-call  VariantControl=(inherit)
      settings: CopyFcn=Stateflow.SLINSF.SimulinkMan.removeBlockPreDeleteFcn  PreDeleteFcn=Stateflow.SLINSF.SimulinkMan.unsafePredeleteFcn
  Chart : Stateflow chart  TreatAsAtomicUnit=on
  FaultType : Outport
  wires:
  Chart/1(FaultType) -> FaultType/1
  ShortGND/1 -> Chart/1(ShortGND)
  Openload/1 -> Chart/2(Openload)

== stateflow chart Appl_HeatFault_CtrlModel/LogicCtrl/HeatDiagnoseCtrl/HeatCommandDeal ==
  state HeatCmd = HeatCmdAquireFunction(API_HeatCmd,HeatCfg,HeatFlg) [function]
  state HeatCmd = HeatCmdAquireFunction1(API_HeatCmd,HeatCfg,HeatFlg) [function]
  state HeatCmd = HeatCmdAquireFunction2(API_HeatCmd,HeatCfg,HeatFlg) [function]
  state DriverHeatCommandDeal [parallel]
    du:
    DrHeatCmd = HeatCmdAquireFunction(HeatFalut_D_SimuIndex_DRHeat,HeatFalut_MemIndexDrHeatConfig,HeatFalut_MemDiagDrHeatFlg);
    settings: executionOrder=1
  state PassengerHeatCommandDeal [parallel]
    du:
    PaHeatCmd = HeatCmdAquireFunction1(HeatFalut_D_SimuIndex_PAHeat,HeatFalut_MemIndexPaHeatConfig,HeatFalut_MemDiagPaHeatFlg);
    settings: executionOrder=2
  state ThirdHeatCommandDeal [parallel]
    du:
    ThirdHeatCmd = HeatCmdAquireFunction2(HeatFalut_D_SimuIndex_ThirdHeat,HeatFalut_MemIndexThirdHeatConfig,TRUE);
    settings: executionOrder=3
  data: API_HeatCmd function_input; HeatCfg function_input; HeatCmd function_output; HeatFlg function_input; API_HeatCmd function_input; HeatCfg function_input; HeatCmd function_output; HeatFlg function_input; API_HeatCmd function_input; HeatCfg function_input; HeatCmd function_output; HeatFlg function_input; HeatFalut_D_SimuIndex_DRHeat input; HeatFalut_D_SimuIndex_PAHeat input; HeatFalut_D_SimuIndex_ThirdHeat input; HeatFalut_MemIndexDrHeatConfig input; HeatFalut_MemIndexPaHeatConfig input; HeatFalut_MemIndexThirdHeatConfig input; DrHeatCmd output uint8; PaHeatCmd output uint8; ThirdHeatCmd output uint8; HeatFalut_MemDiagDrHeatFlg input; HeatFalut_MemDiagPaHeatFlg input; TRUE parameter

== stateflow chart Appl_HeatFault_CtrlModel/LogicCtrl/HeatDiagnoseCtrl/HeatCommandDeal/HeatCmdAquireFunction/HeatCmdAquireFunction ==
  state HeatCmdInvalid
    en:
    HeatCmd = FALSE;
  state HeatCmdValid
    en:
    HeatCmd = TRUE;
  (default) -> HeatCmdInvalid
  HeatCmdInvalid -> HeatCmdValid : /* 指令有效 */
      | [enHeatLvlSts.EN_HEAT_LVL_OFF != API_HeatCmd ...
      | && TRUE == HeatCfg && TRUE == HeatFlg]
  HeatCmdValid -> HeatCmdInvalid : /* 指令无效 */
      | [enHeatLvlSts.EN_HEAT_LVL_OFF == API_HeatCmd ...
      | || TRUE != HeatCfg || TRUE != HeatFlg]
  data: API_HeatCmd input Enum: enHeatLvlSts; HeatCfg input uint8; TRUE parameter; HeatCmd output uint8; FALSE parameter; HeatFlg input uint8

== stateflow chart Appl_HeatFault_CtrlModel/LogicCtrl/HeatDiagnoseCtrl/HeatDiagnoseDeal ==
  state [HeatCmdFault,HeatCmdFault4DTC] = HeatCmdDiagnoseFunction(HeatIOSts,HeatCmd,HeatIS,FaultType) [function]
  state HeatNTCFault = HeatNTCDiagnoseFunction(HeatNTC,NtcMin,NtcMax) [function]
  state [HeatCmdFault,HeatCmdFault4DTC] = HeatCmdDiagnoseFunction1(HeatIOSts,HeatCmd,HeatIS,FaultType) [function]
  state HeatNTCFault = HeatNTCDiagnoseFunction1(HeatNTC,NtcMin,NtcMax) [function]
  state [HeatCmdFault,HeatCmdFault4DTC] = HeatCmdDiagnoseFunction2(HeatIOSts,HeatCmd,HeatIS,FaultType) [function]
  state HeatNTCFault = HeatNTCDiagnoseFunction2(HeatNTC,NtcMin,NtcMax) [function]
  state Driver_HeatDiagnose [parallel]
    du:
    [HeatFault_DRHeatCmdFaultSts,HeatFault_DRHeatCmdFaultSts4DTC] = HeatCmdDiagnoseFunction(HeatFalut_D_SimuIndex_DRHeatIo,DrHeatCmd,HeatFalut_DrHeatIsAdc,DrFaultType);
    HeatFault_DRHeatNTCFaultSts = HeatNTCDiagnoseFunction(HeatFalut_DrHeatNtcAdc,D_HEATFALUT_NtcMin,D_HEATFALUT_NtcMax);
    settings: executionOrder=1
  state Passenger_HeatDiagnose [parallel]
    du:
    [HeatFault_PAHeatCmdFaultSts,HeatFault_PAHeatCmdFaultSts4DTC] = HeatCmdDiagnoseFunction1(HeatFalut_D_SimuIndex_PAHeatIo,PaHeatCmd,HeatFalut_PaHeatIsAdc,PaFaultType);
    HeatFault_PAHeatNTCFaultSts = HeatNTCDiagnoseFunction1(HeatFalut_PaHeatNtcAdc,D_HEATFALUT_NtcMin,D_HEATFALUT_NtcMax);
    settings: executionOrder=2
  state Third_HeatDiagnose [parallel]
    du:
    [HeatFault_ThirdHeatCmdFaultSts,HeatFault_ThirdHeatCmdFaultSts4DTC] = HeatCmdDiagnoseFunction2(HeatFalut_D_SimuIndex_ThirdHeatIo,ThirdHeatCmd,HeatFalut_ThirdHeatIsAdc,ThirdFaultType);
    HeatFault_ThirdHeatNTCFaultSts = HeatNTCDiagnoseFunction2(HeatFalut_ThirdHeatNtcAdc,D_HEATFALUT_NtcMin,D_HEATFALUT_NtcMax);
    settings: executionOrder=3
  data: HeatIOSts function_input; HeatCmd function_input; HeatIS function_input; FaultType function_input; HeatCmdFault function_output; HeatCmdFault4DTC function_output; HeatNTC function_input; HeatNTCFault function_output; NtcMin function_input; NtcMax function_input; HeatIOSts function_input; HeatCmd function_input; HeatIS function_input; FaultType function_input; HeatCmdFault function_output; HeatCmdFault4DTC function_output; HeatNTC function_input; HeatNTCFault function_output; NtcMin function_input; NtcMax function_input; HeatIOSts function_input; HeatCmd function_input; HeatIS function_input; FaultType function_input; HeatCmdFault function_output; HeatCmdFault4DTC function_output; HeatNTC function_input; HeatNTCFault function_output; NtcMin function_input; NtcMax function_input; DrHeatCmd input; PaHeatCmd input; ThirdHeatCmd input; HeatFalut_D_SimuIndex_DRHeatIo input; HeatFalut_D_SimuIndex_PAHeatIo input; HeatFalut_D_SimuIndex_ThirdHeatIo input; HeatFalut_DrHeatNtcAdc input; HeatFalut_PaHeatNtcAdc input; HeatFalut_ThirdHeatNtcAdc input; HeatFalut_DrHeatIsAdc input; HeatFalut_PaHeatIsAdc input; HeatFalut_ThirdHeatIsAdc input; HeatFault_DRHeatCmdFaultSts output Enum: enHeatCmdFault; HeatFault_PAHeatCmdFaultSts output Enum: enHeatCmdFault; HeatFault_ThirdHeatCmdFaultSts output Enum: enHeatCmdFault; HeatFault_DRHeatNTCFaultSts output Enum: enHeatNtcFault; HeatFault_PAHeatNTCFaultSts output Enum: enHeatNtcFault; HeatFault_ThirdHeatNTCFaultSts output Enum: enHeatNtcFault; HeatFault_DRHeatCmdFaultSts4DTC output Enum: enHeatCmdFault; HeatFault_PAHeatCmdFaultSts4DTC output Enum: enHeatCmdFault; HeatFault_ThirdHeatCmdFaultSts4DTC output Enum: enHeatCmdFault; DrFaultType input; PaFaultType input; ThirdFaultType input; D_HEATFALUT_NtcMin parameter; D_HEATFALUT_NtcMax parameter

== stateflow chart Appl_HeatFault_CtrlModel/LogicCtrl/HeatDiagnoseCtrl/HeatDiagnoseDeal/HeatCmdDiagnoseFunction/HeatCmdDiagnose ==
  state HeatCmdDiagnosis
    state CmdShortToGND
      ex:
      ShortTimer = 0;
      (default) -> (junction 25)
      CmdShortToGND -> (junction 25) [order 1]
      (junction 25) -> (junction 28) [order 1] : /* 未超时 */
          | [CAL_CmdShortTime > ShortTimer]
      (junction 25) -> (junction 30) [order 2] : {ShortTimer = CAL_CmdShortTime;
          | HeatCmdFault = enHeatCmdFault.EN_HEAT_FAULT_GND;
          | HeatCmdFault4DTC = enHeatCmdFault.EN_HEAT_FAULT_GND;}
      (junction 28) -> (junction 32) : {ShortTimer++;}
      (junction 32) -> (junction 30)
      (junction 30) -> (junction 35)
    state ShortLow
    state Default
      en:
      OpenTimer = 0;
      ShortTimer = 0;
      HeatCmdFault =  enHeatCmdFault.EN_HEAT_FAULT_NONE;
      RecoverTimer = 0;
      (default) -> (junction 80)
      Default -> (junction 80) [order 1]
      (junction 80) -> (junction 83) [order 1] : /* 未超时 */
          | [CAL_CmdShortTime > RecoverTimer]
      (junction 80) -> (junction 89) [order 2] : {RecoverTimer = CAL_CmdShortTime;
          | HeatCmdFault4DTC =  enHeatCmdFault.EN_HEAT_FAULT_NONE;}
      (junction 83) -> (junction 84) : {RecoverTimer++;}
      (junction 84) -> (junction 89)
      (junction 89) -> (junction 91)
    state CmdOpenLoad
      ex:
      OpenTimer = 0;
      (default) -> (junction 46)
      CmdOpenLoad -> (junction 46) [order 1]
      (junction 46) -> (junction 43) [order 1] : /* 未超时 */
          | [CAL_CmdOpenTime > OpenTimer]
      (junction 46) -> (junction 47) [order 2] : {OpenTimer = CAL_CmdOpenTime;
          | HeatCmdFault = enHeatCmdFault.EN_HEAT_FAULT_OPEN;
          | HeatCmdFault4DTC = enHeatCmdFault.EN_HEAT_FAULT_OPEN;}
      (junction 43) -> (junction 48) : {OpenTimer++;}
      (junction 48) -> (junction 47)
      (junction 47) -> (junction 40)
    state OpenLow
    CmdShortToGND -> ShortLow [order 1] : /* 低电平 */
        | [enHeatIoSts.EN_HEAT_IO_LOW == HeatIOSts]
    ShortLow -> CmdShortToGND : /* 高电平 */
        | [enHeatIoSts.EN_HEAT_IO_HIGH == HeatIOSts]
    (junction 76) -> CmdShortToGND [order 1] : [FaultType == enHeatCmdFault.EN_HEAT_FAULT_GND]
    Default -> CmdShortToGND [order 1] : /* 输出电流对地短路 */
        | [D_HEATFALUT_CmdShortToGnd < HeatIS]
    CmdShortToGND -> Default [order 2] : /* 输出电流对地短路恢复 */
        | [D_HEATFALUT_CmdShortToGnd >= HeatIS]
    CmdOpenLoad -> CmdShortToGND [order 3] : /* 输出电流对地短路 */
        | [D_HEATFALUT_CmdShortToGnd < HeatIS]
    CmdShortToGND -> CmdOpenLoad [order 3] : /* 输出电流开路 */
        | [D_HEATFALUT_CmdOpenLoad > HeatIS]
    (default) -> (junction 76)
    (junction 76) -> Default [order 3]
    (junction 76) -> CmdOpenLoad [order 2] : [FaultType == enHeatCmdFault.EN_HEAT_FAULT_OPEN]
    Default -> CmdOpenLoad [order 2] : /* 输出电流开路 */
        | [D_HEATFALUT_CmdOpenLoad > HeatIS]
    CmdOpenLoad -> Default [order 2] : /* 输出电流开路恢复 */
        | [D_HEATFALUT_CmdOpenLoad <= HeatIS]
    CmdOpenLoad -> OpenLow [order 1] : /* 低电平 */
        | [enHeatIoSts.EN_HEAT_IO_LOW == HeatIOSts]
    OpenLow -> CmdOpenLoad : /* 高电平 */
        | [enHeatIoSts.EN_HEAT_IO_HIGH == HeatIOSts]
  state HeatCmdClose
    en:
    OpenTimer = 0;
    ShortTimer = 0;
    HeatCmdFault = enHeatCmdFault.EN_HEAT_FAULT_NONE;
    ex:
    HeatCmdFault4DTC = FaultType;
  (default) -> HeatCmdClose
  HeatCmdClose -> HeatCmdDiagnosis : /* 加热CMD */
      | [TRUE == HeatCmd]
  HeatCmdDiagnosis -> HeatCmdClose : /* 无加热CMD */
      | [TRUE != HeatCmd]
  data: HeatIOSts input Enum: enHeatIoSts; HeatCmd input uint8; HeatIS input uint16; HeatCmdFault output Enum: enHeatCmdFault; ShortTimer local uint8; OpenTimer local uint8; CAL_CmdShortTime parameter; CAL_CmdOpenTime parameter; D_HEATFALUT_CmdShortToGnd parameter; D_HEATFALUT_CmdOpenLoad parameter; TRUE parameter; HeatCmdFault4DTC output Enum: enHeatCmdFault; FaultType input; RecoverTimer local uint8

== stateflow chart Appl_HeatFault_CtrlModel/LogicCtrl/HeatDiagnoseCtrl/HeatDiagnoseDeal/HeatNTCDiagnoseFunction/HeatCmdDiagnose ==
  state NTCShortToGND
    ex:
    ShortTimer = 0;
    (default) -> (junction 77)
    NTCShortToGND -> (junction 77) [order 1]
    (junction 77) -> (junction 80) [order 1] : /* 短地超时 */
        | [CAL_NTCShortTime > ShortTimer]
    (junction 77) -> (junction 82) [order 2] : {ShortTimer = CAL_NTCShortTime;
        | HeatNTCFault = enHeatNtcFault.EN_NTC_FAULT_GND;}
    (junction 80) -> (junction 84) : {ShortTimer++;}
    (junction 84) -> (junction 82)
    (junction 82) -> (junction 87)
  state Default
    en:
    WaitAquireTimer = 1;
    RecoveryTimer = 0;
    ex:
    WaitAquireTimer = 0;
    (default) -> (junction 64)
    (junction 64) -> (junction 69) [order 1] : /* 等待超时 */
        | [CAL_NTCWaitTime  > WaitAquireTimer]
    Default -> (junction 64) [order 1]
    (junction 69) -> (junction 71) : {WaitAquireTimer ++;}
    (junction 64) -> (junction 67) [order 2] : {WaitAquireTimer = CAL_NTCWaitTime;}
    (junction 71) -> (junction 67)
    (junction 67) -> (junction 74)
    (junction 74) -> (junction 139) [order 1] : [HeatNTCFault != enHeatNtcFault.EN_NTC_FAULT_NONE]
    (junction 74) -> (junction 162) [order 2]
    (junction 139) -> (junction 141) : {RecoveryTimer++; }
    (junction 141) -> (junction 143) [order 1] : /* NTC不可信故障*/
        | [HeatNTCFault == enHeatNtcFault.EN_NTC_FAULT_UNC]
    (junction 143) -> (junction 145) [order 1] : [/*计时超过5s*/
        | CAL_NTCOverTime < RecoveryTimer]
    (junction 141) -> (junction 152) [order 2]
    (junction 143) -> (junction 158) [order 2]
    (junction 145) -> (junction 150) : {RecoveryTimer = CAL_NTCOverTime;
        | HeatNTCFault = enHeatNtcFault.EN_NTC_FAULT_NONE;}
    (junction 152) -> (junction 154) [order 1] : [/*开路和短地时间皆为1s*/
        | CAL_NTCOpenTime < RecoveryTimer]
    (junction 152) -> (junction 160) [order 2]
    (junction 154) -> (junction 156) : {RecoveryTimer = CAL_NTCOpenTime;
        | HeatNTCFault = enHeatNtcFault.EN_NTC_FAULT_NONE;}
    (junction 162) -> (junction 160)
    (junction 156) -> (junction 160)
    (junction 158) -> (junction 156)
    (junction 150) -> (junction 158)
    (junction 160) -> (junction 168)
  state NTCOpenLoad
    ex:
    OpenTimer = 0;
    (default) -> (junction 94)
    NTCOpenLoad -> (junction 94) [order 1]
    (junction 94) -> (junction 92) [order 1] : /* 开路超时 */
        | [CAL_NTCOpenTime  > OpenTimer]
    (junction 94) -> (junction 95) [order 2] : {OpenTimer = CAL_NTCOpenTime;
        | HeatNTCFault = enHeatNtcFault.EN_NTC_FAULT_OPEN;}
    (junction 92) -> (junction 97) : {OpenTimer ++;}
    (junction 97) -> (junction 95)
    (junction 95) -> (junction 100)
  state NTCOverRange
    ex:
    OverTimer = 0;
    (default) -> (junction 105)
    NTCOverRange -> (junction 105) [order 1]
    (junction 105) -> (junction 108) [order 1] : /* 不可信超时 */
        | [CAL_NTCOverTime   > OverTimer]
    (junction 105) -> (junction 109) [order 2] : {OverTimer = CAL_NTCOverTime ;
        | HeatNTCFault = enHeatNtcFault.EN_NTC_FAULT_UNC;}
    (junction 108) -> (junction 110) : {OverTimer ++;}
    (junction 110) -> (junction 109)
    (junction 109) -> (junction 112)
  NTCShortToGND -> Default [order 1] : /* 对地短路 */
      | [D_HEATFALUT_NtcShortToGnd < HeatNTC]
  Default -> NTCShortToGND [order 1] : /* 对地恢复 */
      | [D_HEATFALUT_NtcShortToGnd >= HeatNTC ...
      | && CAL_NTCWaitTime <= WaitAquireTimer]
  (default) -> Default
  Default -> NTCOpenLoad [order 2] : /* NTC开路 */
      | [D_HEATFALUT_NtcOpenLoad < HeatNTC ...
      | && CAL_NTCWaitTime <= WaitAquireTimer]
  NTCOpenLoad -> Default [order 1] : /* NTC开路恢复*/
      | [D_HEATFALUT_NtcOpenLoad >= HeatNTC]
  Default -> NTCOverRange [order 3] : /* NTC 不可信 */
      | [(NtcMax < HeatNTC ...
      | || NtcMin > HeatNTC) ...
      | && CAL_NTCWaitTime <= WaitAquireTimer]
  NTCOverRange -> Default [order 1] : /* NTC不可信恢复 */
      | [(NtcMax >= HeatNTC && NtcMin <= HeatNTC) ...
      | || D_HEATFALUT_NtcOpenLoad < HeatNTC ...
      | || D_HEATFALUT_NtcShortToGnd >= HeatNTC]
  data: HeatNTC input uint16; HeatNTCFault output Enum: enHeatNtcFault; ShortTimer local uint16; WaitAquireTimer local uint16; OpenTimer local uint16; OverTimer local uint16; CAL_NTCOpenTime parameter; CAL_NTCOverTime parameter; CAL_NTCShortTime parameter; CAL_NTCWaitTime parameter; D_HEATFALUT_NtcOpenLoad parameter; D_HEATFALUT_NtcShortToGnd parameter; RecoveryTimer local uint16; NtcMin input uint16; NtcMax input uint16

== stateflow chart Appl_HeatFault_CtrlModel/LogicCtrl/HeatDiagnoseCtrl/HeatCommandDeal/HeatCmdAquireFunction1/HeatCmdAquireFunction ==
  state HeatCmdInvalid
    en:
    HeatCmd = FALSE;
  state HeatCmdValid
    en:
    HeatCmd = TRUE;
  (default) -> HeatCmdInvalid
  HeatCmdInvalid -> HeatCmdValid : /* 指令有效 */
      | [enHeatLvlSts.EN_HEAT_LVL_OFF != API_HeatCmd ...
      | && TRUE == HeatCfg && TRUE == HeatFlg]
  HeatCmdValid -> HeatCmdInvalid : /* 指令无效 */
      | [enHeatLvlSts.EN_HEAT_LVL_OFF == API_HeatCmd ...
      | || TRUE != HeatCfg || TRUE != HeatFlg]
  data: API_HeatCmd input Enum: enHeatLvlSts; HeatCfg input uint8; TRUE parameter; HeatCmd output uint8; FALSE parameter; HeatFlg input uint8

== stateflow chart Appl_HeatFault_CtrlModel/LogicCtrl/HeatDiagnoseCtrl/HeatCommandDeal/HeatCmdAquireFunction2/HeatCmdAquireFunction ==
  state HeatCmdInvalid
    en:
    HeatCmd = FALSE;
  state HeatCmdValid
    en:
    HeatCmd = TRUE;
  (default) -> HeatCmdInvalid
  HeatCmdInvalid -> HeatCmdValid : /* 指令有效 */
      | [enHeatLvlSts.EN_HEAT_LVL_OFF != API_HeatCmd ...
      | && TRUE == HeatCfg && TRUE == HeatFlg]
  HeatCmdValid -> HeatCmdInvalid : /* 指令无效 */
      | [enHeatLvlSts.EN_HEAT_LVL_OFF == API_HeatCmd ...
      | || TRUE != HeatCfg || TRUE != HeatFlg]
  data: API_HeatCmd input Enum: enHeatLvlSts; HeatCfg input uint8; TRUE parameter; HeatCmd output uint8; FALSE parameter; HeatFlg input uint8

== stateflow chart Appl_HeatFault_CtrlModel/LogicCtrl/HeatDiagnoseCtrl/HeatDiagnoseDeal/HeatCmdDiagnoseFunction1/HeatCmdDiagnose ==
  state HeatCmdDiagnosis
    state CmdShortToGND
      ex:
      ShortTimer = 0;
      (default) -> (junction 25)
      CmdShortToGND -> (junction 25) [order 1]
      (junction 25) -> (junction 28) [order 1] : /* 未超时 */
          | [CAL_CmdShortTime > ShortTimer]
      (junction 25) -> (junction 30) [order 2] : {ShortTimer = CAL_CmdShortTime;
          | HeatCmdFault = enHeatCmdFault.EN_HEAT_FAULT_GND;
          | HeatCmdFault4DTC = enHeatCmdFault.EN_HEAT_FAULT_GND;}
      (junction 28) -> (junction 32) : {ShortTimer++;}
      (junction 32) -> (junction 30)
      (junction 30) -> (junction 35)
    state ShortLow
    state Default
      en:
      OpenTimer = 0;
      ShortTimer = 0;
      HeatCmdFault =  enHeatCmdFault.EN_HEAT_FAULT_NONE;
      RecoverTimer = 0;
      (default) -> (junction 80)
      Default -> (junction 80) [order 1]
      (junction 80) -> (junction 83) [order 1] : /* 未超时 */
          | [CAL_CmdShortTime > RecoverTimer]
      (junction 80) -> (junction 89) [order 2] : {RecoverTimer = CAL_CmdShortTime;
          | HeatCmdFault4DTC =  enHeatCmdFault.EN_HEAT_FAULT_NONE;}
      (junction 83) -> (junction 84) : {RecoverTimer++;}
      (junction 84) -> (junction 89)
      (junction 89) -> (junction 91)
    state CmdOpenLoad
      ex:
      OpenTimer = 0;
      (default) -> (junction 46)
      CmdOpenLoad -> (junction 46) [order 1]
      (junction 46) -> (junction 43) [order 1] : /* 未超时 */
          | [CAL_CmdOpenTime > OpenTimer]
      (junction 46) -> (junction 47) [order 2] : {OpenTimer = CAL_CmdOpenTime;
          | HeatCmdFault = enHeatCmdFault.EN_HEAT_FAULT_OPEN;
          | HeatCmdFault4DTC = enHeatCmdFault.EN_HEAT_FAULT_OPEN;}
      (junction 43) -> (junction 48) : {OpenTimer++;}
      (junction 48) -> (junction 47)
      (junction 47) -> (junction 40)
    state OpenLow
    CmdShortToGND -> ShortLow [order 1] : /* 低电平 */
        | [enHeatIoSts.EN_HEAT_IO_LOW == HeatIOSts]
    ShortLow -> CmdShortToGND : /* 高电平 */
        | [enHeatIoSts.EN_HEAT_IO_HIGH == HeatIOSts]
    (junction 76) -> CmdShortToGND [order 1] : [FaultType == enHeatCmdFault.EN_HEAT_FAULT_GND]
    Default -> CmdShortToGND [order 1] : /* 输出电流对地短路 */
        | [D_HEATFALUT_CmdShortToGnd < HeatIS]
    CmdShortToGND -> Default [order 2] : /* 输出电流对地短路恢复 */
        | [D_HEATFALUT_CmdShortToGnd >= HeatIS]
    CmdOpenLoad -> CmdShortToGND [order 3] : /* 输出电流对地短路 */
        | [D_HEATFALUT_CmdShortToGnd < HeatIS]
    CmdShortToGND -> CmdOpenLoad [order 3] : /* 输出电流开路 */
        | [D_HEATFALUT_CmdOpenLoad > HeatIS]
    (default) -> (junction 76)
    (junction 76) -> Default [order 3]
    (junction 76) -> CmdOpenLoad [order 2] : [FaultType == enHeatCmdFault.EN_HEAT_FAULT_OPEN]
    Default -> CmdOpenLoad [order 2] : /* 输出电流开路 */
        | [D_HEATFALUT_CmdOpenLoad > HeatIS]
    CmdOpenLoad -> Default [order 2] : /* 输出电流开路恢复 */
        | [D_HEATFALUT_CmdOpenLoad <= HeatIS]
    CmdOpenLoad -> OpenLow [order 1] : /* 低电平 */
        | [enHeatIoSts.EN_HEAT_IO_LOW == HeatIOSts]
    OpenLow -> CmdOpenLoad : /* 高电平 */
        | [enHeatIoSts.EN_HEAT_IO_HIGH == HeatIOSts]
  state HeatCmdClose
    en:
    OpenTimer = 0;
    ShortTimer = 0;
    HeatCmdFault = enHeatCmdFault.EN_HEAT_FAULT_NONE;
    ex:
    HeatCmdFault4DTC = FaultType;
  (default) -> HeatCmdClose
  HeatCmdClose -> HeatCmdDiagnosis : /* 加热CMD */
      | [TRUE == HeatCmd]
  HeatCmdDiagnosis -> HeatCmdClose : /* 无加热CMD */
      | [TRUE != HeatCmd]
  data: HeatIOSts input Enum: enHeatIoSts; HeatCmd input uint8; HeatIS input uint16; HeatCmdFault output Enum: enHeatCmdFault; ShortTimer local uint8; OpenTimer local uint8; CAL_CmdShortTime parameter; CAL_CmdOpenTime parameter; D_HEATFALUT_CmdShortToGnd parameter; D_HEATFALUT_CmdOpenLoad parameter; TRUE parameter; HeatCmdFault4DTC output Enum: enHeatCmdFault; FaultType input; RecoverTimer local uint8
